simulink model "XunJi_PID"  (Simulink 9.0)
settings: Solver=FixedStepAuto  StartTime=0.0  StopTime=100  FixedStep=0.01  RelTol=1e-3
InitFcn:
  | kp=100
  | ki=50
  | kd=0
  | pre_x=5
libraries: Solver_SF x1
settings Model: LogicAnalyzerSignalOrdering=2aae8837-395f-4747-809b-cd8f96e4e84d  Creator=yinch  LastModifiedBy=yinch
settings DataIOCC: SaveFormat=Dataset
settings OptimizationCC: LifeSpan=auto
settings DebuggingCC: UnderspecifiedInitializationDetection=Simplified  MergeDetectMultiDrivingBlocksExec=error  SFUnexpectedBacktrackingDiag=error  SFNoUnconditionalDefaultTransitionDiag=error  SFExecutionAtInitializationDiag=warning
settings HardwareCC: ProdBitPerPointer=64  ProdBitPerSizeT=64  ProdBitPerPtrDiffT=64  ProdLargestAtomicFloat=Float  ProdIntDivRoundTo=Zero  ProdEndianess=LittleEndian  ProdWordSize=64  ProdHWDeviceType=Intel->x86-64 (Windows64)
settings ModelReferenceCC: PropagateSignalLabelsOutOfModel=on
settings CodeAppCC: StateflowObjectComments=off
settings GRTTargetCC: TargetLangStandard=C99 (ISO)
settings ConfigComp: CovMetricSettings=dwe  CovHtmlReporting=off  CovSaveCumulativeToWorkspaceVar=off  CovSaveSingleToWorkspaceVar=off  CovExternalEMLEnable=on

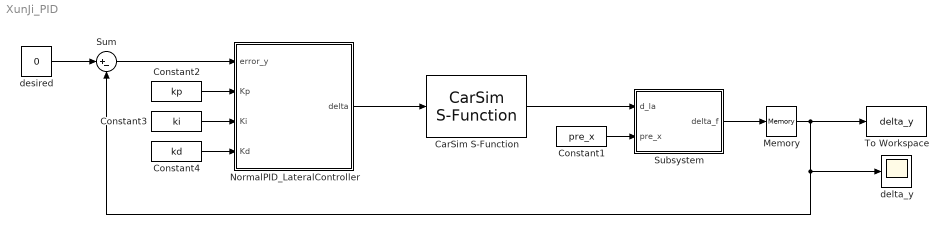
== system XunJi_PID ==
  CarSim S-Function : Solver_SF/CarSim S-Function  Priority=1  VehicleCode=i_i  SIMFILE=simfile
  Constant1 : Constant  Value=pre_x
  Constant2 : Constant  Value=kp
  Constant3 : Constant  Value=ki
  Constant4 : Constant  Value=kd
  Memory : Memory
  NormalPID_LateralController : Subsystem
  Subsystem : Subsystem
  Sum : Sum  Inputs=|+-
  To Workspace : ToWorkspace  VariableName=delta_y  SampleTime=-1
  delta_y : Scope
  desired : Constant  Value=0
  wires:
  desired/1 -> Sum/1
  Memory/1 -> delta_y/1, Sum/2, To Workspace/1
  Sum/1 -> NormalPID_LateralController/1(error_y)
  NormalPID_LateralController/1(delta) -> CarSim S-Function/1
  CarSim S-Function/1 -> Subsystem/1(d_la)
  Constant1/1 -> Subsystem/2(pre_x)
  Subsystem/1(delta_f) -> Memory/1
  Constant2/1 -> NormalPID_LateralController/2(Kp)
  Constant3/1 -> NormalPID_LateralController/3(Ki)
  Constant4/1 -> NormalPID_LateralController/4(Kd)

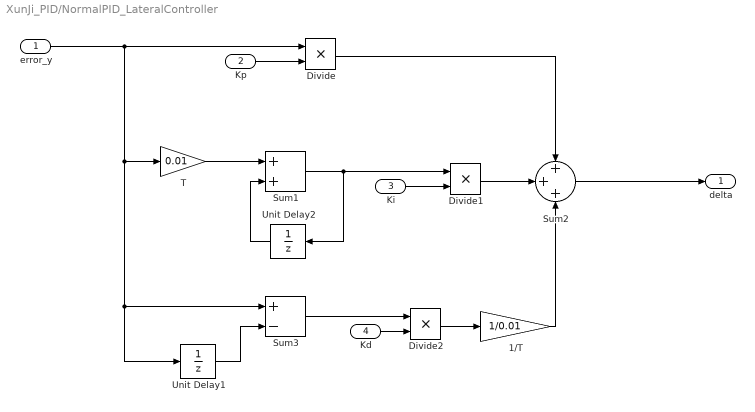
== system XunJi_PID/NormalPID_LateralController ==
  error_y : Inport
  Kp : Inport  Port=2
  Ki : Inport  Port=3
  Kd : Inport  Port=4
  1/T : Gain  Gain=1/0.01
  Divide : Product  Inputs=**
  Divide1 : Product  Inputs=**
  Divide2 : Product  Inputs=**
  Sum1 : Sum
  Sum2 : Sum  Inputs=+++
  Sum3 : Sum  Inputs=+-
  T : Gain  Gain=0.01
  Unit Delay1 : UnitDelay  SampleTime=-1
  Unit Delay2 : UnitDelay  SampleTime=-1
  delta : Outport
  wires:
  Sum2/1 -> delta/1
  Kp/1 -> Divide/2
  error_y/1 -> Unit Delay1/1, Sum3/1, T/1, Divide/1
  Divide/1 -> Sum2/1
  T/1 -> Sum1/1
  Sum1/1 -> Unit Delay2/1, Divide1/1
  Divide1/1 -> Sum2/2
  Ki/1 -> Divide1/2
  Unit Delay2/1 -> Sum1/2
  Unit Delay1/1 -> Sum3/2
  Sum3/1 -> Divide2/1
  Kd/1 -> Divide2/2
  Divide2/1 -> 1/T/1
  1/T/1 -> Sum2/3

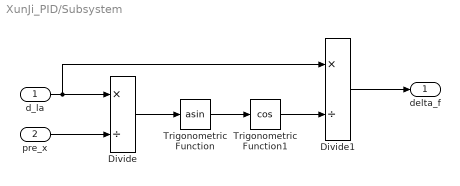
== system XunJi_PID/Subsystem ==
  d_la : Inport
  pre_x : Inport  Port=2
  Divide : Product  Inputs=*/
  Divide1 : Product  Inputs=*/
  Trigonometric Function : Trigonometry  Operator=asin
  Trigonometric Function1 : Trigonometry  Operator=cos
  delta_f : Outport
  wires:
  Trigonometric Function1/1 -> Divide1/2
  Divide1/1 -> delta_f/1
  Divide/1 -> Trigonometric Function/1
  d_la/1 -> Divide1/1, Divide/1
  pre_x/1 -> Divide/2
  Trigonometric Function/1 -> Trigonometric Function1/1
